simulink model "stm32f4_timerirq_demo"  (Simulink 7.3)
settings: Solver=ode3  SolverMode=SingleTasking  StartTime=0.0  StopTime=10.0  RelTol=1e-3
PreLoadFcn:
  | waijung.modelPreload; % Required for working with Waijung Blockset. Do not remove.
undefined symbols (not defined in the file): HSEOSC, Link, LQFP176, ST, STM32F417IG
libraries: stm32f4_io_lib x4, stm32f4_tim_lib x4, stm32f4_device_config_lib x1
CloseFcn:
  | waijung.modelClose; % Required for working with Waijung Blockset. Do not remove.
settings Model: Creator=Krisada  LastModifiedBy=Krisada
settings OptimizationCC: OptimizeModelRefInitCode=on  LifeSpan=1
settings HardwareCC: ProdEndianess=LittleEndian  ProdHWDeviceType=ARM Compatible->Cortex - M4  TargetEndianess=LittleEndian  TargetHWDeviceType=ARM Compatible->Cortex - M4
settings RTWCC: SystemTargetFile=stm32f4.tlc  GenerateMakefile=off  TemplateMakefile=ert_default_tmf  Description=STM32F4 Target  ProcessScript=stm32f4_make_rtw_hook
settings CodeAppCC: IgnoreCustomStorageClasses=off
settings STFCustomTargetCC: ModelReferenceCompliant=off  CombineOutputUpdateFcns=on  ERTCustomFileBanners=on  SupportContinuousTime=off  SupportNonInlinedSFcns=off  SystemTargetFile=stm32f4.tlc
settings ERTTargetCC: MultiwordLength=2048  ModelReferenceCompliant=off  ParMdlRefBuildCompliant=off  CompOptLevelCompliant=off  ERTFirstTimeCompliant=off  ModelStepFunctionPrototypeControlCompliant=off  CPPClassGenCompliant=off  InlinedParameterPlacement=NonHierarchical  ERTSrcFileBannerTemplate=stm32f4_code_template.cgt  ERTHdrFileBannerTemplate=stm32f4_code_template.cgt  ERTDataSrcFileTemplate=stm32f4_code_template.cgt  ERTDataHdrFileTemplate=stm32f4_code_template.cgt  ERTCustomFileTemplate=stm32f4_file_process.tlc

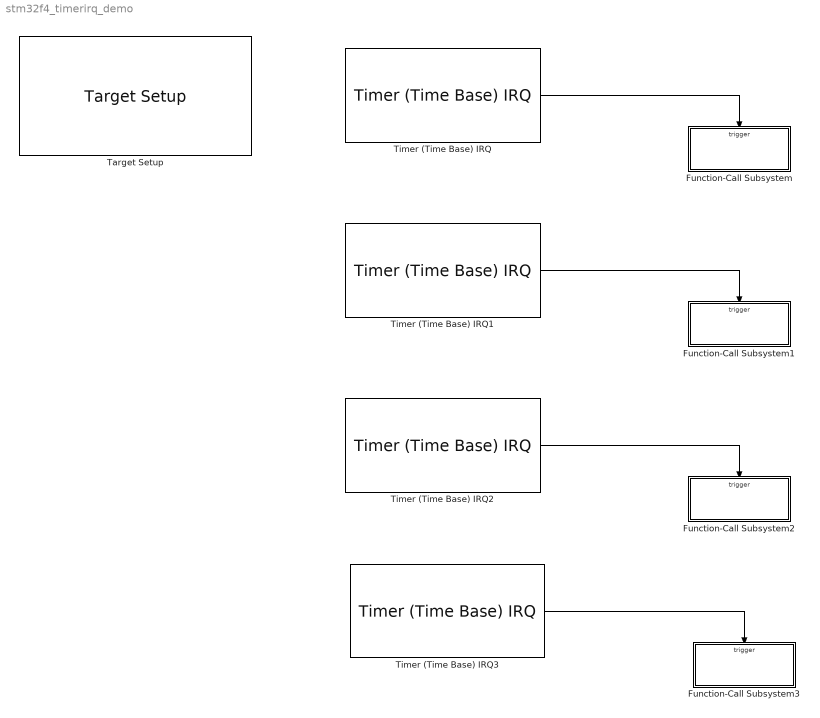
== system stm32f4_timerirq_demo ==
  Function-Call Subsystem : Subsystem  TreatAsAtomicUnit=on
  Function-Call Subsystem1 : Subsystem  TreatAsAtomicUnit=on
  Function-Call Subsystem2 : Subsystem  TreatAsAtomicUnit=on
  Function-Call Subsystem3 : Subsystem  TreatAsAtomicUnit=on
  Target Setup : stm32f4_device_config_lib/Target Setup  Priority=100  compiler=GNU ARM  previous_compiler=GNU ARM  mcu=STM32F417IG (LQFP176)  mcustr=STM32F417IG  clockconfig=HSEOSC-8MHz  system_stm32f4xx_c_path=F:\trunk\targets\stm32f4_target\stm32f4\utils\system_stm32f4xx_default\STM32F40_41xxx\hseosc8mhz  showmemoryconfiguration=off  stacksize=0x400  heapsize=0x200  enableautocompiledownload=on  fullchiperase=off  programmerinterface=ST-Link  editctrlstr=on  compilercontrolstr=$(patsubst %, -I%, .) -mcpu=cortex-m4 -mthumb -mthumb-interwork -mfloat-abi=hard -mfpu=fpv4-sp-d16 -ffast-math -Wall -Wextra -Ofast  assemblercontrolstr=$(patsubst %, -I%, .) -mcpu=cortex-m4 -mthumb -mthumb-interwork -mfloat-abi=hard -mfpu=fpv4-sp-d16 -ffast-math -Wall -Wextra -Ofast -Wa,-amhls=$(<:.s=.lst) -D__STACK_SIZE=$(STACK_SIZE) -D__HEAP_SIZE=$(HEAP_SIZE)  linkercontrolstr=-T$(LD_SCRIPT) -g -Wl,-Map=$(MAP),--cref,--no-warn-mismatch -mcpu=cortex-m4 -mthumb -mthumb-interwork -mfloat-abi=hard -mfpu=fpv4-sp-d16 -specs=nosys.specs  runafterdownload=on  execprofile=None  profileruart=1  profilerbaud=115200  profilertxpin=D8  profilerinitstr=0.01,168000000,1680000,115200,0  manualsetsampletime=off  sampletime=0.01  blockid=TargetSetup  systickreloadvalue=1680000  hseval=8000000  lastprofileruart=1  hclk=168000000  flashorigin=0x8000000  flashlength=1024k  ramorigin=0x20000000  ramlength=128k  useextram=off
  Timer (Time Base) IRQ : stm32f4_tim_lib/Timer (Time Base) IRQ  configmode=Basic  timer=2  nvicprioritygroup=4  irqpreemptionpriority_g0=0  irqpreemptionpriority_g1=0  irqpreemptionpriority_g2=0  irqpreemptionpriority_g3=4  irqpreemptionpriority_g4=0  irqpreemptionpriority=0  irqsubpriority_g0=0  irqsubpriority_g1=0  irqsubpriority_g2=0  irqsubpriority_g3=0  irqsubpriority_g4=0  irqsubpriority=0  sampletime=1  autoreload=65521  prescaler=1281  blockid=TimerTimeBaseIRQ
  Timer (Time Base) IRQ1 : stm32f4_tim_lib/Timer (Time Base) IRQ  configmode=Basic  timer=3  nvicprioritygroup=4  irqpreemptionpriority_g0=0  irqpreemptionpriority_g1=0  irqpreemptionpriority_g2=0  irqpreemptionpriority_g3=4  irqpreemptionpriority_g4=0  irqpreemptionpriority=0  irqsubpriority_g0=0  irqsubpriority_g1=0  irqsubpriority_g2=0  irqsubpriority_g3=0  irqsubpriority_g4=0  irqsubpriority=0  sampletime=2  autoreload=65521  prescaler=2563  blockid=TimerTimeBaseIRQ1
  Timer (Time Base) IRQ2 : stm32f4_tim_lib/Timer (Time Base) IRQ  configmode=Basic  timer=4  nvicprioritygroup=4  irqpreemptionpriority_g0=0  irqpreemptionpriority_g1=0  irqpreemptionpriority_g2=0  irqpreemptionpriority_g3=4  irqpreemptionpriority_g4=0  irqpreemptionpriority=0  irqsubpriority_g0=0  irqsubpriority_g1=0  irqsubpriority_g2=0  irqsubpriority_g3=0  irqsubpriority_g4=0  irqsubpriority=0  sampletime=3  autoreload=65521  prescaler=3845  blockid=TimerTimeBaseIRQ2
  Timer (Time Base) IRQ3 : stm32f4_tim_lib/Timer (Time Base) IRQ  configmode=Basic  timer=5  nvicprioritygroup=4  irqpreemptionpriority_g0=0  irqpreemptionpriority_g1=0  irqpreemptionpriority_g2=0  irqpreemptionpriority_g3=4  irqpreemptionpriority_g4=0  irqpreemptionpriority=0  irqsubpriority_g0=0  irqsubpriority_g1=0  irqsubpriority_g2=0  irqsubpriority_g3=0  irqsubpriority_g4=0  irqsubpriority=0  sampletime=4  autoreload=65534  prescaler=5126  blockid=TimerTimeBaseIRQ3
  wires:
  Timer (Time Base) IRQ/1 -> Function-Call Subsystem/Trigger
  Timer (Time Base) IRQ1/1 -> Function-Call Subsystem1/Trigger
  Timer (Time Base) IRQ2/1 -> Function-Call Subsystem2/Trigger
  Timer (Time Base) IRQ3/1 -> Function-Call Subsystem3/Trigger

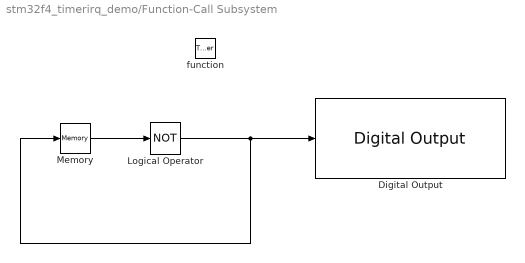
== system stm32f4_timerirq_demo/Function-Call Subsystem ==
  function : TriggerPort  TriggerType=function-call
  Digital Output : stm32f4_io_lib/Digital Output  use_bitband=on  port=D  speed=100  porttype=Push Pull  porttypestr=PP  use_pin0=off  use_pin1=off  use_pin2=off  use_pin3=off  use_pin4=off  use_pin5=off  use_pin6=off  use_pin7=off  use_pin8=off  use_pin9=off  use_pin10=off  use_pin11=off  use_pin12=on  use_pin13=off  use_pin14=off  use_pin15=off  pinstr=GPIO_Pin_12  usedpinarray="[0  0  0  0  0  0  0  0  0  0  0  0  1  0  0  0]"  bitbandingstr="#define FunctionCallSubsystemDigitalOutput_D12 Peripheral_BB(GPIOD->ODR, 12)  /* Output pin */"  sampletime=-1  sampletimestr=-1  blockid=FunctionCallSubsystemDigitalOutput  enablecustomportlabel=off  globalinit=off  cinputportlabel=In1, In2  coutputportlabel=0
  Logical Operator : Logic  Operator=NOT  AllPortsSameDT=off  OutDataTypeMode=boolean  LogicDataType=fixdt(0, 8)  OutDataTypeStr=boolean
  Memory : Memory  InheritSampleTime=on
  wires:
  Memory/1 -> Logical Operator/1
  Logical Operator/1 -> Digital Output/1, Memory/1

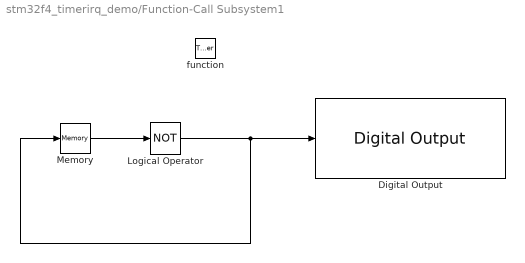
== system stm32f4_timerirq_demo/Function-Call Subsystem1 ==
  function : TriggerPort  TriggerType=function-call
  Digital Output : stm32f4_io_lib/Digital Output  use_bitband=on  port=D  speed=100  porttype=Push Pull  porttypestr=PP  use_pin0=off  use_pin1=off  use_pin2=off  use_pin3=off  use_pin4=off  use_pin5=off  use_pin6=off  use_pin7=off  use_pin8=off  use_pin9=off  use_pin10=off  use_pin11=off  use_pin12=off  use_pin13=on  use_pin14=off  use_pin15=off  pinstr=GPIO_Pin_13  usedpinarray="[0  0  0  0  0  0  0  0  0  0  0  0  0  1  0  0]"  bitbandingstr="#define FunctionCallSubsystem1DigitalOutput_D13 Peripheral_BB(GPIOD->ODR, 13)  /* Output pin */"  sampletime=-1  sampletimestr=-1  blockid=FunctionCallSubsystem1DigitalOutput  enablecustomportlabel=off  globalinit=off  cinputportlabel=In1, In2  coutputportlabel=0
  Logical Operator : Logic  Operator=NOT  AllPortsSameDT=off  OutDataTypeMode=boolean  LogicDataType=fixdt(0, 8)  OutDataTypeStr=boolean
  Memory : Memory  InheritSampleTime=on
  wires:
  Logical Operator/1 -> Memory/1, Digital Output/1
  Memory/1 -> Logical Operator/1

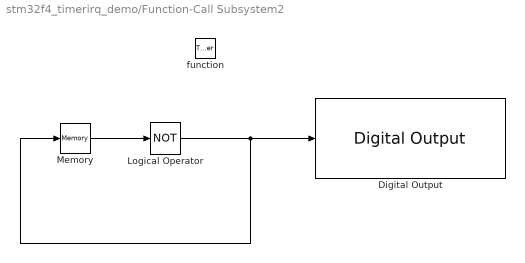
== system stm32f4_timerirq_demo/Function-Call Subsystem2 ==
  function : TriggerPort  TriggerType=function-call
  Digital Output : stm32f4_io_lib/Digital Output  use_bitband=on  port=D  speed=100  porttype=Push Pull  porttypestr=PP  use_pin0=off  use_pin1=off  use_pin2=off  use_pin3=off  use_pin4=off  use_pin5=off  use_pin6=off  use_pin7=off  use_pin8=off  use_pin9=off  use_pin10=off  use_pin11=off  use_pin12=off  use_pin13=off  use_pin14=on  use_pin15=off  pinstr=GPIO_Pin_14  usedpinarray="[0  0  0  0  0  0  0  0  0  0  0  0  0  0  1  0]"  bitbandingstr="#define FunctionCallSubsystem2DigitalOutput_D14 Peripheral_BB(GPIOD->ODR, 14)  /* Output pin */"  sampletime=-1  sampletimestr=-1  blockid=FunctionCallSubsystem2DigitalOutput  enablecustomportlabel=off  globalinit=off  cinputportlabel=In1, In2  coutputportlabel=0
  Logical Operator : Logic  Operator=NOT  AllPortsSameDT=off  OutDataTypeMode=boolean  LogicDataType=fixdt(0, 8)  OutDataTypeStr=boolean
  Memory : Memory  InheritSampleTime=on
  wires:
  Memory/1 -> Logical Operator/1
  Logical Operator/1 -> Digital Output/1, Memory/1

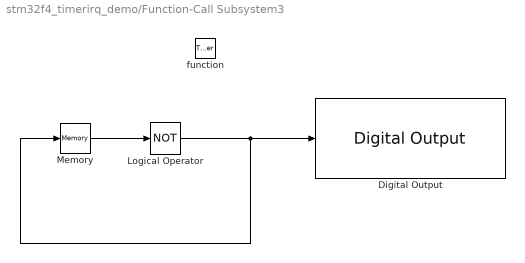
== system stm32f4_timerirq_demo/Function-Call Subsystem3 ==
  function : TriggerPort  TriggerType=function-call
  Digital Output : stm32f4_io_lib/Digital Output  use_bitband=on  port=D  speed=100  porttype=Push Pull  porttypestr=PP  use_pin0=off  use_pin1=off  use_pin2=off  use_pin3=off  use_pin4=off  use_pin5=off  use_pin6=off  use_pin7=off  use_pin8=off  use_pin9=off  use_pin10=off  use_pin11=off  use_pin12=off  use_pin13=off  use_pin14=off  use_pin15=on  pinstr=GPIO_Pin_15  usedpinarray="[0  0  0  0  0  0  0  0  0  0  0  0  0  0  0  1]"  bitbandingstr="#define FunctionCallSubsystem3DigitalOutput_D15 Peripheral_BB(GPIOD->ODR, 15)  /* Output pin */"  sampletime=-1  sampletimestr=-1  blockid=FunctionCallSubsystem3DigitalOutput  enablecustomportlabel=off  globalinit=off  cinputportlabel=In1, In2  coutputportlabel=0
  Logical Operator : Logic  Operator=NOT  AllPortsSameDT=off  OutDataTypeMode=boolean  LogicDataType=fixdt(0, 8)  OutDataTypeStr=boolean
  Memory : Memory  InheritSampleTime=on
  wires:
  Logical Operator/1 -> Memory/1, Digital Output/1
  Memory/1 -> Logical Operator/1
